simulink model "first_task"  (R2023a)
settings: Solver=VariableStepAuto  StartTime=0.0  StopTime=Tdes  RelTol=1e-3
undefined symbols (not defined in the file): alpha0, ke, kq, s_sw, vs_des, x0, y0
settings Model: Creator=Nabil Samaan  LastModifiedBy=dvogureckiy99
settings DebuggingCC: UnconnectedInputMsg=warning  UnconnectedOutputMsg=warning  UnconnectedLineMsg=warning
settings ModelReferenceCC: EnableRefExpFcnMdlSchedulingChecks=on
settings RTWCC: DLArmComputeVersion=19.05

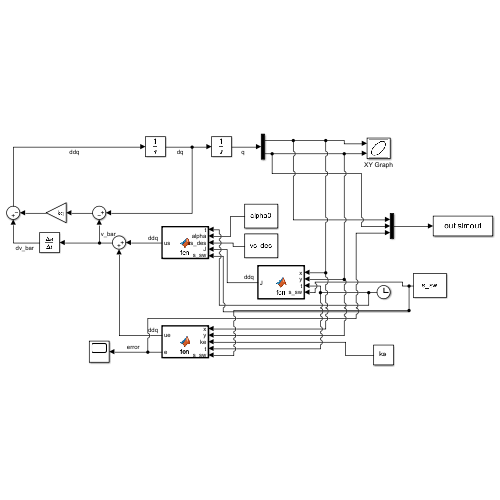
[thumbnail: Simulink's stored preview of the top-level diagram]
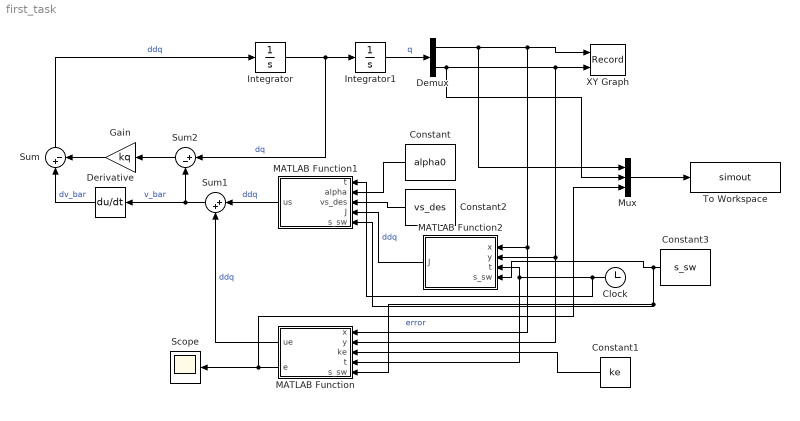
== system first_task ==
  Clock : Clock
  Constant : Constant  Value=alpha0
  Constant1 : Constant  Value=ke
  Constant2 : Constant  Value=vs_des
  Constant3 : Constant  Value=s_sw
  Demux : Demux  Outputs=2
  Derivative : Derivative  CoefficientInTFapproximation=0.001
  Gain : Gain  Gain=kq
  Integrator : Integrator
  Integrator1 : Integrator  InitialCondition=[x0;y0]
  MATLAB Function : MATLAB Function  TreatAsAtomicUnit=on
  MATLAB Function1 : MATLAB Function  TreatAsAtomicUnit=on
  MATLAB Function2 : MATLAB Function  TreatAsAtomicUnit=on
  Mux : Mux  Inputs=3
  Scope : Scope
  Sum : Sum  Inputs=|+-
  Sum1 : Sum  Inputs=|++
  Sum2 : Sum  Inputs=|+-
  To Workspace : ToWorkspace  VariableName=simout  SampleTime=-1
  XY Graph : Record  FileSettingsInternal="{\"entries\":[{\"content\":{\"excelSettings\":{\"content\":{},\"type\":\"Streamout.ExcelSettings\"}},\"type\":\"Streamout.FileSettingStorage\",\"uuid\":\"\"}],\"packageUris\":[\"http:\\/\\/schema.mathworks.com\\/mf0\\/streamout_blocks\\/R2020a\"],\"version\":\"1.0\"}"  Layout=[1 1]  SignalsInternal="{\"entries\":[{\"content\":{\"signals\":[{\"content\":{\"blockPath\":[],\"dimensions\":[1,1],\"domain\":\"\",\"lineColor\":\"#a2142f\",\"plots\":[1],\"port\":1,\"sid\":[\"\"],\"signalID\":3168,\"signalName\":\"Demux:1\"},\"type\":\"RecordBlkView.Signal\",\"uuid\":\"\"},{\"content\":{\"blockPath\":[],\"dimensions\":[1,1],\"domain\":\"\",\"lineColor\":\"#139fff\",\"plots\":[1],\"port\":2,\"sid\":[\"\"],\"signalID\":3172,\"signalName\":\"Demux:2\"},\"type\":\"RecordBlkView.Signal\",\"uuid\":\"\"}]},\"type\":\"RecordBlkView.InputSignals\",\"uuid\":\"\"}],\"packageUris\":[\"http:\\/\\/schema.mathworks.com\\/mf0\\/streamout_blocks\\/R2020a\"],\"version\":\"1.0\"}"  VisualizationBindings="{\"xyplotplugin\":{\"info\":[{\"series\":[{\"bindingParametersList\":[{\"parameter\":\"X-Axis\",\"signalID\":3168,\"signalName\":\"Demux:1\"},{\"parameter\":\"Y-Axis\",\"signalID\":3172,\"signalName\":\"Demux:2\"}],\"seriesID\":21916}],\"subplotID\":1}]}}"  CompatibilityTag=XY
  wires:
  Demux/1 -> Mux/1, XY Graph/1, MATLAB Function/1(x), MATLAB Function2/1(x)
  Demux/2 -> Mux/2, XY Graph/2, MATLAB Function/2(y), MATLAB Function2/2(y)
  Integrator/1 -> Sum2/1, Integrator1/1  "dq"
  Integrator1/1 -> Demux/1  "q"
  Sum/1 -> Integrator/1  "ddq"
  MATLAB Function2/1(J) -> MATLAB Function1/4(J)  "ddq"
  Constant/1 -> MATLAB Function1/2(alpha)
  Constant1/1 -> MATLAB Function/3(ke)
  MATLAB Function1/1(us) -> Sum1/1  "ddq"
  MATLAB Function/1(ue) -> Sum1/2  "ddq"
  Sum1/1 -> Derivative/1, Sum2/2  "v_bar"
  Sum2/1 -> Gain/1
  Gain/1 -> Sum/2
  Derivative/1 -> Sum/1  "dv_bar"
  Constant2/1 -> MATLAB Function1/3(vs_des)
  Clock/1 -> MATLAB Function1/1(t), MATLAB Function/4(t), MATLAB Function2/3(t)
  MATLAB Function/2(e) -> Mux/3, Scope/1  "error"
  Mux/1 -> To Workspace/1
  Constant3/1 -> MATLAB Function1/5(s_sw), MATLAB Function/5(s_sw), MATLAB Function2/4(s_sw)

== matlab function first_task/MATLAB Function1 ==
  data: t input; alpha input; vs_des input; J input; us output; s_sw input
function us = fcn(t,alpha, vs_des, J,s_sw)

R=[cos(alpha) sin(alpha); -sin(alpha) cos(alpha)];

if t>s_sw(1) && t<s_sw(2) 
    vs_des = -vs_des;
end
us=R*(J^(-1))*[vs_des;0];

== matlab function first_task/MATLAB Function ==
  data: x input; ue output; y input; ke input; t input; e output; s_sw input
function [ue,e] = fcn(x,y,ke,t,s_sw)

if(t<=s_sw(1))
    ue=-ke* ( ((x+3)^2+(y-2)^2-9)*[2*x+6;2*y-4]);
    e=((x+3)^2+(y-2)^2-9);
elseif(t<=s_sw(2))
    ue=-ke*(y-2*cos(0.5*x+0.3)-2)*[sin(0.5*x+0.3);1];
    e=(y-2*cos(0.5*x+0.3)-2);
else
    ue=-ke*((x-12)^2+(y-2)^2-25)*[2*x-24;2*y-4];
    e=((x-12)^2+(y-2)^2-25);
end

== matlab function first_task/MATLAB Function2 ==
  data: x input; J output; y input; t input; s_sw input
function J = fcn(x,y,t,s_sw)

if (t<=s_sw(1))
    J=[2*y-4,-2*x-6;2*x+6,2*y-4];
elseif(t<=s_sw(2)) 
    J=[1,-sin(0.5*x+0.3);sin(0.5*x+0.3),1];
else
    J=[2*y-4,24-2*x;2*x-24,2*y-4];
end
